simulink model "buck_averaged"  (R2024b)
settings: Solver=VariableStepAuto  StartTime=0.0  StopTime=.02  RelTol=1e-3
undefined symbols (not defined in the file): D
settings Model: Creator=luisg  LastModifiedBy=luisg
settings DataIOCC: ReturnWorkspaceOutputs=off

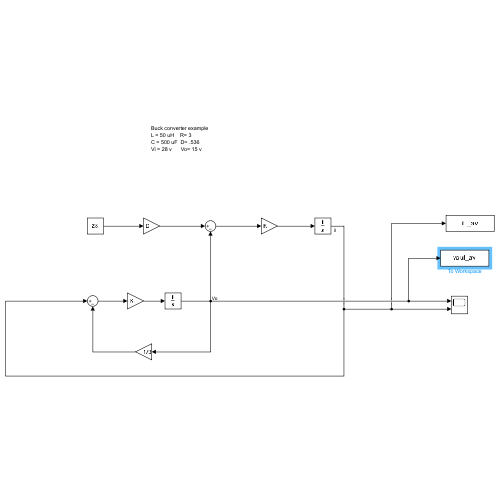
[thumbnail: Simulink's stored preview of the top-level diagram]
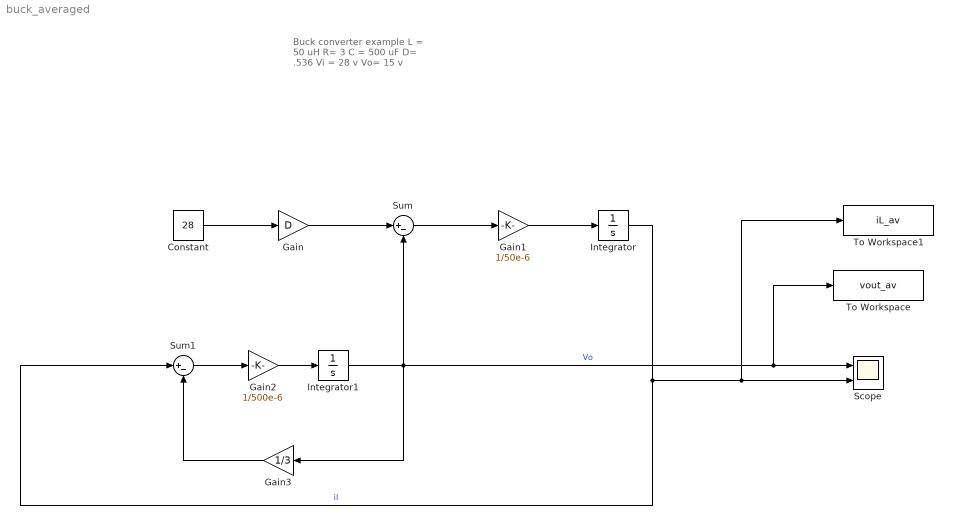
== system buck_averaged ==
  note: Buck converter example
      | L = 50 uH    R= 3
      | C = 500 uF  D= .536
      | Vi = 28 v      Vo= 15 v
  Constant : Constant  Value=28
  Gain : Gain  Gain=D
  Gain1 : Gain  Gain=1/50e-6
  Gain2 : Gain  Gain=1/500e-6
  Gain3 : Gain  Gain=1/3
  Integrator : Integrator
  Integrator1 : Integrator
  Scope : Scope  NumInputPorts=2
  Sum : Sum  Inputs=|+-
  Sum1 : Sum  Inputs=|+-
  To Workspace : ToWorkspace  VariableName=vout_av  SaveFormat=Structure With Time  SampleTime=-1
  To Workspace1 : ToWorkspace  VariableName=iL_av  SaveFormat=Structure With Time  SampleTime=-1
  wires:
  Constant/1 -> Gain/1
  Gain/1 -> Sum/1
  Sum/1 -> Gain1/1
  Gain1/1 -> Integrator/1
  Sum1/1 -> Gain2/1
  Gain2/1 -> Integrator1/1
  Integrator1/1 -> To Workspace/1, Scope/1, Sum/2, Gain3/1  "Vo"
  Integrator/1 -> To Workspace1/1, Scope/2, Sum1/1  "il"
  Gain3/1 -> Sum1/2
